simulink model "SF009A_DutyCycThermProtn"  (R2013b)
settings: Solver=FixedStepDiscrete  SolverMode=SingleTasking  StartTime=0.0  StopTime=1  FixedStep=0.1  RelTol=1e-3
undefined symbols (not defined in the file): AbsltTThermLimCnt, ARCHGLBPRM_100MILLISEC_SEC_F32, CTRLRANDCUTFLT_CNT_U08, CTRLRTFLT_CNT_U08, CUTFLT_CNT_U08, DITHERMLIM_MOTNWTMTR_F32, DutyCycExcddCnt, DutyCycThermProtnAbsltCtrlTTblX, DutyCycThermProtnAbsltCtrlTTqTblY, DutyCycThermProtnAbsltCuTTblX, DutyCycThermProtnAbsltCuTTqTblY, DutyCycThermProtnAbsltMotVelBreakPt, DutyCycThermProtnAbsltTTqSlewHiLim, DutyCycThermProtnAbsltTTqSlewLoLim, DutyCycThermProtnCtrlT, DutyCycThermProtnCtrlTSeln, DutyCycThermProtnDutyCycFildThd, DutyCycThermProtnIgnOffCtrlEna, DutyCycThermProtnIgnOffMsgWaitTi, DutyCycThermProtnLstTblValNonStall, DutyCycThermProtnLstTblValStall, DutyCycThermProtnMotPrTSeln, DutyCycThermProtnMplr1NonStallTblY, DutyCycThermProtnMplr1StallTblY, DutyCycThermProtnMplr2NonStallTblY, DutyCycThermProtnMplr2StallTblY, DutyCycThermProtnMplr3NonStallTblY, DutyCycThermProtnMplr3StallTblY, DutyCycThermProtnMplr4NonStallTblY, DutyCycThermProtnMplr4StallTblY, DutyCycThermProtnMplr5NonStallTblY, DutyCycThermProtnMplr5StallTblY, DutyCycThermProtnMplr6NonStallTblY, DutyCycThermProtnMplr6StallTblY, DutyCycThermProtnMplrTblX, DutyCycThermProtnMplrTSeln, DutyCycThermProtnSlowFilTSeln, DutyCycThermProtnThermLoadLimTblX, DutyCycThermProtnThermLoadLimTblY, DutyCycThermProtnTqCmdSlewDwn, DutyCycThermProtnTqCmdSlewUp, FILVALMIN_ULS_F32, IGNTIOFFTHD_CNT_F32, NODEBSTEP_CNT_U16, NtcSts1, NvmGetErrSts1, ONEPERC_ULS_F32, TAU3_SEC_F32, TAU4_SEC_F32, TAU5_SEC_F32, TAU6_SEC_F32, THERMLOADLIMTBLIDX_ULS_U08
libraries: FixdToFloat x13, Fil x12, simulink x11, NxtrLim x10, NxtrMath x8, FloatToFixd x6, NxtrMax x6, NxtrMin x4, NxtrAbslt x2, NxtrNvM x1
(part 3 of 6)

== system SF009A_DutyCycThermProtn/DutyCycThermProtn/DutyCycThermProtnInit1/PowerOnTasks/DefaultIgnOffTime ==
  Action Port : ActionPort  ActionType=else
  CopyRight2 : Subsystem  Description=|  mask(Copyright Information){none=on}
      | Copyright info block.                                               
      |                                                                     
      | Place copyright information at the top of every subsystem in design.
      mask prompts: none "No parameters"
      mask help: Place copyright information at the top of every subsystem in design.
      mask Display:
      | NxtrConf = 'Nexteer Confidential';
      | 
      | sys = bdroot; %handle for the current model ("system")
      | first = get_param(sys,'Created');
      | first = first(end-3:end);  %year is last four digits
      | 
      | last = get_param(sys,'LastModifiedDate');
      | if isempty(last)
      |     last = datestr(now,'yyyy');
      | else
      |     last = last(end-3:end);
      | end
      | 
      | if strcmp(first,last)
      |     fprintf('%s -- Copyright %s Nexteer',NxtrConf,first)
      | else
      |     fprintf('%s -- %s%s- %s Nexteer',NxtrConf,char(169),first,last)
      | end
  DefIgnOffTime1 : Constant  RequirementInfo="{'linktype_rmi_doors' '0000a52a (/E-STEER Core/SubSystem Specifications/Application Functions/SF009A Thermal Duty Cycle Protection)' '#SF009A_285' 'true' 'REQ:  SF009A_285' '' } %GIDa_1c1a8355_68c4_4a16_a698_2c7b860aa81f"  Value=FILVALMIN_ULS_F32
  FiltSV3 : Outport  RequirementInfo="{'linktype_rmi_doors' '0000a52a (/E-STEER Core/SubSystem Specifications/Application Functions/SF009A Thermal Duty Cycle Protection)' '#SF009A_285' 'true' 'REQ:  SF009A_285' '' } %GIDa_f53f9a1c_8faf_4833_a80c_e2891c436a6f"
  FiltSV4 : Outport  RequirementInfo="{'linktype_rmi_doors' '0000a52a (/E-STEER Core/SubSystem Specifications/Application Functions/SF009A Thermal Duty Cycle Protection)' '#SF009A_285' 'true' 'REQ:  SF009A_285' '' } %GIDa_7573da05_c607_444c_bff7_05b9be356769"  Port=2
  FiltSV5 : Outport  RequirementInfo="{'linktype_rmi_doors' '0000a52a (/E-STEER Core/SubSystem Specifications/Application Functions/SF009A Thermal Duty Cycle Protection)' '#SF009A_285' 'true' 'REQ:  SF009A_285' '' } %GIDa_0a22d052_a9b5_4254_83f4_8f154e55c7ba"  Port=3
  FiltSV6 : Outport  RequirementInfo="{'linktype_rmi_doors' '0000a52a (/E-STEER Core/SubSystem Specifications/Application Functions/SF009A Thermal Duty Cycle Protection)' '#SF009A_285' 'true' 'REQ:  SF009A_285' '' } %GIDa_7f0b1c6f_6523_47e0_8553_42c05ca6b0db"  Port=4
  wires:
  DefIgnOffTime1/1 -> FiltSV3/1, FiltSV4/1, FiltSV6/1, FiltSV5/1

== system SF009A_DutyCycThermProtn/DutyCycThermProtn/DutyCycThermProtnInit1/PowerOnTasks/InputIgnOffTime ==
  note: RANGE CHECK, ENSURE VALUE IS BELOW A CONSTANT (10000)
  IgnTiOff : Inport
  Action Port : ActionPort  ActionType=then
  CopyRight2 : Subsystem  Description=|  mask(Copyright Information){none=on}
      | Copyright info block.                                               
      |                                                                     
      | Place copyright information at the top of every subsystem in design.
      mask prompts: none "No parameters"
      mask help: Place copyright information at the top of every subsystem in design.
      mask Display:
      | NxtrConf = 'Nexteer Confidential';
      | 
      | sys = bdroot; %handle for the current model ("system")
      | first = get_param(sys,'Created');
      | first = first(end-3:end);  %year is last four digits
      | 
      | last = get_param(sys,'LastModifiedDate');
      | if isempty(last)
      |     last = datestr(now,'yyyy');
      | else
      |     last = last(end-3:end);
      | end
      | 
      | if strcmp(first,last)
      |     fprintf('%s -- Copyright %s Nexteer',NxtrConf,first)
      | else
      |     fprintf('%s -- %s%s- %s Nexteer',NxtrConf,char(169),first,last)
      | end
  Data Store Read : DataStoreRead  DataStoreName=FilStVal  DataStoreElements=FilStVal.Fil3StVal
  Data Store Read1 : DataStoreRead  DataStoreName=FilStVal  DataStoreElements=FilStVal.Fil4StVal
  Data Store Read2 : DataStoreRead  DataStoreName=FilStVal  DataStoreElements=FilStVal.Fil5StVal
  Data Store Read3 : DataStoreRead  DataStoreName=FilStVal  DataStoreElements=FilStVal.Fil6StVal
  Filt3ExpDecay : Subsystem  RequirementInfo={} %GIDa_9f9f3f65_c145_44e4_82e5_fd713760ae68
  Filt4ExpDecay : Subsystem  RequirementInfo={} %GIDa_626963e8_8ecf_441f_b1c9_4240579d77f9
  Filt5ExpDecay : Subsystem  RequirementInfo={} %GIDa_9364c89b_18fa_4473_8499_21374c540da9
  Filt6ExpDecay : Subsystem  RequirementInfo={} %GIDa_8e6049b9_bd81_40a5_96f3_6037c184dcb3
  FiltSV3 : Outport
  FiltSV4 : Outport  Port=2
  FiltSV5 : Outport  Port=3
  FiltSV6 : Outport  Port=4
  wires:
  Filt3ExpDecay/1(FiltSV) -> FiltSV3/1
  Data Store Read/1 -> Filt3ExpDecay/2(FiltSVOrg)
  Filt4ExpDecay/1(FiltSV) -> FiltSV4/1
  Filt5ExpDecay/1(FiltSV) -> FiltSV5/1
  Data Store Read2/1 -> Filt5ExpDecay/2(FiltSVOrg)
  Filt6ExpDecay/1(FiltSV) -> FiltSV6/1
  Data Store Read3/1 -> Filt6ExpDecay/2(FiltSVOrg)
  Data Store Read1/1 -> Filt4ExpDecay/2(FiltSVOrg)
  IgnTiOff/1 -> Filt3ExpDecay/1(IgnTimeOffSel), Filt4ExpDecay/1(IgnTimeOffSel), Filt6ExpDecay/1(IgnTimeOffSel), Filt5ExpDecay/1(IgnTimeOffSel)

== system SF009A_DutyCycThermProtn/DutyCycThermProtn/DutyCycThermProtnInit1/SetInitialValueOfAbsTempLimitSlew/Copyright1 ==

== system SF009A_DutyCycThermProtn/DutyCycThermProtn/DutyCycThermProtnInit1/SetInitialValueOfLstTblValRateLimrStVari/Copyright1 ==

== system SF009A_DutyCycThermProtn/DutyCycThermProtn/DutyCycThermProtnPer1/FiltSVReinit/CopyRight2 ==

== system SF009A_DutyCycThermProtn/DutyCycThermProtn/DutyCycThermProtnPer1/FiltSVReinit/VehTiVldDisabled ==
  Action Port : ActionPort  ActionType=else
  CopyRight2 : Subsystem  Description=|  mask(Copyright Information){none=on}
      | Copyright info block.                                               
      |                                                                     
      | Place copyright information at the top of every subsystem in design.
      mask prompts: none "No parameters"
      mask help: Place copyright information at the top of every subsystem in design.
      mask Display:
      | NxtrConf = 'Nexteer Confidential';
      | 
      | sys = bdroot; %handle for the current model ("system")
      | first = get_param(sys,'Created');
      | first = first(end-3:end);  %year is last four digits
      | 
      | last = get_param(sys,'LastModifiedDate');
      | if isempty(last)
      |     last = datestr(now,'yyyy');
      | else
      |     last = last(end-3:end);
      | end
      | 
      | if strcmp(first,last)
      |     fprintf('%s -- Copyright %s Nexteer',NxtrConf,first)
      | else
      |     fprintf('%s -- %s%s- %s Nexteer',NxtrConf,char(169),first,last)
      | end
  DefIgnOffTime1 : Constant  RequirementInfo="{'linktype_rmi_doors' '0000a52a (/E-STEER Core/SubSystem Specifications/Application Functions/SF009A Thermal Duty Cycle Protection)' '#SF009A_285' 'true' 'REQ:  SF009A_285' '' } %GIDa_ff571b1a_1782_4f5b_8061_ceec6519b3d1"  Value=FILVALMIN_ULS_F32
  FiltSV3 : Outport  RequirementInfo="{'linktype_rmi_doors' '0000a52a (/E-STEER Core/SubSystem Specifications/Application Functions/SF009A Thermal Duty Cycle Protection)' '#SF009A_285' 'true' 'REQ:  SF009A_285' '' } %GIDa_7dd21f81_ccc7_49b6_9939_90cfad62de91"
  FiltSV4 : Outport  RequirementInfo="{'linktype_rmi_doors' '0000a52a (/E-STEER Core/SubSystem Specifications/Application Functions/SF009A Thermal Duty Cycle Protection)' '#SF009A_285' 'true' 'REQ:  SF009A_285' '' } %GIDa_9e3d7e87_4137_4c20_943f_e98c68156777"  Port=2
  FiltSV5 : Outport  RequirementInfo="{'linktype_rmi_doors' '0000a52a (/E-STEER Core/SubSystem Specifications/Application Functions/SF009A Thermal Duty Cycle Protection)' '#SF009A_285' 'true' 'REQ:  SF009A_285' '' } %GIDa_7d2d2855_4602_487a_979b_6bffe0216b93"  Port=3
  FiltSV6 : Outport  RequirementInfo="{'linktype_rmi_doors' '0000a52a (/E-STEER Core/SubSystem Specifications/Application Functions/SF009A Thermal Duty Cycle Protection)' '#SF009A_285' 'true' 'REQ:  SF009A_285' '' } %GIDa_d4f64410_e786_41b0_841d_daea9815ca41"  Port=4
  wires:
  DefIgnOffTime1/1 -> FiltSV3/1, FiltSV4/1, FiltSV6/1, FiltSV5/1

== system SF009A_DutyCycThermProtn/DutyCycThermProtn/DutyCycThermProtnPer1/FiltSVReinit/VehTiVldEnabled ==
  IgnTiOff : Inport
  Action Port : ActionPort  ActionType=then
  CopyRight2 : Subsystem  Description=|  mask(Copyright Information){none=on}
      | Copyright info block.                                               
      |                                                                     
      | Place copyright information at the top of every subsystem in design.
      mask prompts: none "No parameters"
      mask help: Place copyright information at the top of every subsystem in design.
      mask Display:
      | NxtrConf = 'Nexteer Confidential';
      | 
      | sys = bdroot; %handle for the current model ("system")
      | first = get_param(sys,'Created');
      | first = first(end-3:end);  %year is last four digits
      | 
      | last = get_param(sys,'LastModifiedDate');
      | if isempty(last)
      |     last = datestr(now,'yyyy');
      | else
      |     last = last(end-3:end);
      | end
      | 
      | if strcmp(first,last)
      |     fprintf('%s -- Copyright %s Nexteer',NxtrConf,first)
      | else
      |     fprintf('%s -- %s%s- %s Nexteer',NxtrConf,char(169),first,last)
      | end
  Data Store Read : DataStoreRead  DataStoreName=Fil3ValPwrUp
  Data Store Read1 : DataStoreRead  DataStoreName=Fil4ValPwrUp
  Data Store Read2 : DataStoreRead  DataStoreName=Fil5ValPwrUp
  Data Store Read3 : DataStoreRead  DataStoreName=Fil6ValPwrUp
  Filt3ExpDecay : Subsystem
  Filt4ExpDecay : Subsystem
  Filt5ExpDecay : Subsystem
  Filt6ExpDecay : Subsystem
  FiltSV3 : Outport
  FiltSV4 : Outport  Port=2
  FiltSV5 : Outport  Port=3
  FiltSV6 : Outport  Port=4
  wires:
  IgnTiOff/1 -> Filt6ExpDecay/1(IgnTimeOffSel), Filt5ExpDecay/1(IgnTimeOffSel), Filt4ExpDecay/1(IgnTimeOffSel), Filt3ExpDecay/1(IgnTimeOffSel)
  Data Store Read3/1 -> Filt6ExpDecay/2(FiltSVOrg)
  Filt6ExpDecay/1(FiltSV) -> FiltSV6/1
  Data Store Read2/1 -> Filt5ExpDecay/2(FiltSVOrg)
  Filt5ExpDecay/1(FiltSV) -> FiltSV5/1
  Data Store Read1/1 -> Filt4ExpDecay/2(FiltSVOrg)
  Filt4ExpDecay/1(FiltSV) -> FiltSV4/1
  Data Store Read/1 -> Filt3ExpDecay/2(FiltSVOrg)
  Filt3ExpDecay/1(FiltSV) -> FiltSV3/1

== system SF009A_DutyCycThermProtn/DutyCycThermProtn/DutyCycThermProtnPer1/LoadLimiting/CopyRight2 ==

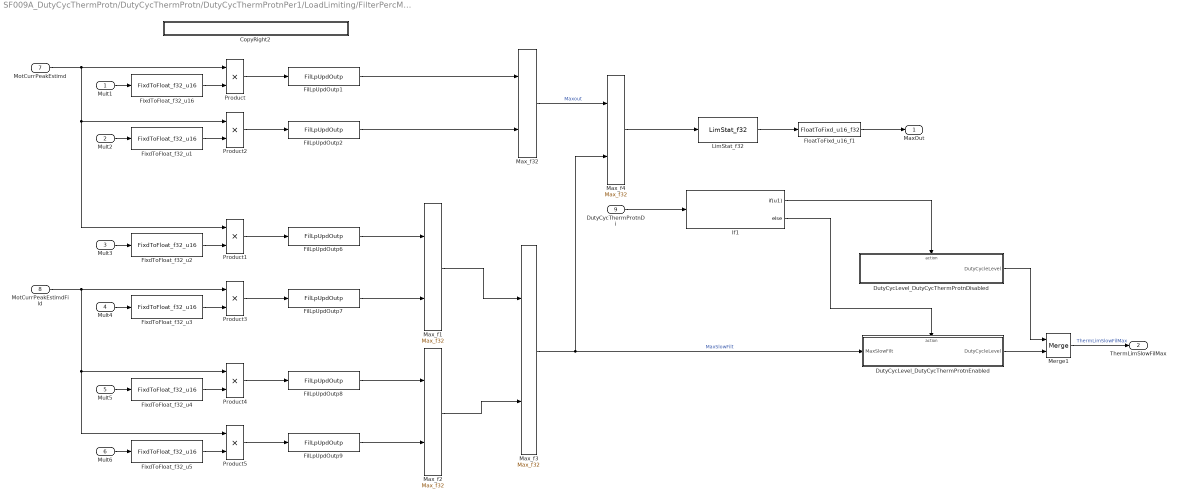
== system SF009A_DutyCycThermProtn/DutyCycThermProtn/DutyCycThermProtnPer1/LoadLimiting/FilterPercMax ==
  Mult1 : Inport
  Mult2 : Inport  Port=2
  Mult3 : Inport  Port=3
  Mult4 : Inport  Port=4
  Mult5 : Inport  Port=5
  Mult6 : Inport  Port=6
  MotCurrPeakEstimd : Inport  Port=7
  MotCurrPeakEstimdFild : Inport  Port=8
  DutyCycThermProtnDi : Inport  Port=9
  CopyRight2 : Subsystem  Description=|  mask(Copyright Information){none=on}
      | Copyright info block.                                               
      |                                                                     
      | Place copyright information at the top of every subsystem in design.
      mask prompts: none "No parameters"
      mask help: Place copyright information at the top of every subsystem in design.
      mask Display:
      | NxtrConf = 'Nexteer Confidential';
      | 
      | sys = bdroot; %handle for the current model ("system")
      | first = get_param(sys,'Created');
      | first = first(end-3:end);  %year is last four digits
      | 
      | last = get_param(sys,'LastModifiedDate');
      | if isempty(last)
      |     last = datestr(now,'yyyy');
      | else
      |     last = last(end-3:end);
      | end
      | 
      | if strcmp(first,last)
      |     fprintf('%s -- Copyright %s Nexteer',NxtrConf,first)
      | else
      |     fprintf('%s -- %s%s- %s Nexteer',NxtrConf,char(169),first,last)
      | end
  DutyCycLevel_DutyCycThermProtnDisabled : Subsystem  RequirementInfo="{'linktype_rmi_doors' '0000a52a (/E-STEER Core/SubSystem Specifications/Application Functions/SF009A Thermal Duty Cycle Protection)' '#SF009A_168' 'true' 'REQ:  SF009A_168' '' } %GIDa_71363024_cb12_46dd_971c_3c161e9d529d"  TreatAsAtomicUnit=on
  DutyCycLevel_DutyCycThermProtnEnabled : Subsystem  RequirementInfo="{'linktype_rmi_doors' '0000a52a (/E-STEER Core/SubSystem Specifications/Application Functions/SF009A Thermal Duty Cycle Protection)' '#SF009A_168' 'true' 'REQ:  SF009A_168' '' } %GIDa_1862e0cc_48c0_4a64_b3aa_9ef2fa11f229"  TreatAsAtomicUnit=on
  FilLpUpdOutp1 : Fil/FilLpUpdOutp  RequirementInfo="{'linktype_rmi_doors' '0000a52a (/E-STEER Core/SubSystem Specifications/Application Functions/SF009A Thermal Duty Cycle Protection)' '#SF009A_117' 'true' 'REQ:  SF009A_117' '' } %GIDa_36d69916_80a2_4684_8052_fd4d54618007"  StVar=Fil1ValStVari
      settings: AttributesFormatString=StVar: %<StVar>
  FilLpUpdOutp2 : Fil/FilLpUpdOutp  RequirementInfo="{'linktype_rmi_doors' '0000a52a (/E-STEER Core/SubSystem Specifications/Application Functions/SF009A Thermal Duty Cycle Protection)' '#SF009A_117' 'true' 'REQ:  SF009A_117' '' } %GIDa_9334f7f9_570f_473a_a841_bd6f3c21f9df"  StVar=Fil2ValStVari
      settings: AttributesFormatString=StVar: %<StVar>
  FilLpUpdOutp6 : Fil/FilLpUpdOutp  RequirementInfo="{'linktype_rmi_doors' '0000a52a (/E-STEER Core/SubSystem Specifications/Application Functions/SF009A Thermal Duty Cycle Protection)' '#SF009A_117' 'true' 'REQ:  SF009A_117' '' } %GIDa_8cd640f7_4fe0_46fd_98bb_13b2eab9fb91"  StVar=Fild3Val
      settings: AttributesFormatString=StVar: %<StVar>
  FilLpUpdOutp7 : Fil/FilLpUpdOutp  RequirementInfo="{'linktype_rmi_doors' '0000a52a (/E-STEER Core/SubSystem Specifications/Application Functions/SF009A Thermal Duty Cycle Protection)' '#SF009A_117' 'true' 'REQ:  SF009A_117' '' } %GIDa_84154e02_2e1c_41ac_9811_25a1fbb85ef4"  StVar=Fild4Val
      settings: AttributesFormatString=StVar: %<StVar>
  FilLpUpdOutp8 : Fil/FilLpUpdOutp  RequirementInfo="{'linktype_rmi_doors' '0000a52a (/E-STEER Core/SubSystem Specifications/Application Functions/SF009A Thermal Duty Cycle Protection)' '#SF009A_117' 'true' 'REQ:  SF009A_117' '' } %GIDa_4a9913a0_954a_4382_b1cf_522ede446f9f"  StVar=Fild5Val
      settings: AttributesFormatString=StVar: %<StVar>
  FilLpUpdOutp9 : Fil/FilLpUpdOutp  RequirementInfo="{'linktype_rmi_doors' '0000a52a (/E-STEER Core/SubSystem Specifications/Application Functions/SF009A Thermal Duty Cycle Protection)' '#SF009A_117' 'true' 'REQ:  SF009A_117' '' } %GIDa_c55f5e10_5865_48ee_8ffc_2f75da5ed5de"  StVar=Fild6Val
      settings: AttributesFormatString=StVar: %<StVar>
  FixdToFloat_f32_u{1..5,16} (6 alike) : FixdToFloat/FixdToFloat_f32_u16  Param1=13
  FloatToFixd_u16_f1 : FloatToFixd/FloatToFixd_u16_f32  Param1=0
  If1 : If  RequirementInfo="{'linktype_rmi_doors' '0000a52a (/E-STEER Core/SubSystem Specifications/Application Functions/SF009A Thermal Duty Cycle Protection)' '#SF009A_168' 'true' 'REQ:  SF009A_168' '' } %GIDa_157cb9dd_8c28_4ea7_a2f6_9f40ccd5ede0"  IfExpression=u1
  LimStat_f32 : NxtrLim/LimStat_f32  LoLim=single(0)  HiLim=FILOUTPLIM_ULS_F32
      settings: AttributesFormatString=Lower Limit: %<LoLim>\nUpper Limit: %<HiLim>
  Max_f1 : NxtrMax/Max_f32  RequirementInfo="{'linktype_rmi_doors' '0000a52a (/E-STEER Core/SubSystem Specifications/Application Functions/SF009A Thermal Duty Cycle Protection)' '#SF009A_164' 'true' 'REQ:  SF009A_164' '' ; 'linktype_rmi_doors' '0000a52a (/E-STEER Core/SubSystem Specifications/Application Functions/SF009A Thermal Duty Cycle Protection)' '#SF009A_167' 'true' 'REQ:  SF009A_167' '' } %GIDa_ca8925de_f515_4e09_b430_d40efee02347"  SFunctionSpec=single y1 = Max_f32(single u1, single u2)
  Max_f2 : NxtrMax/Max_f32  RequirementInfo="{'linktype_rmi_doors' '0000a52a (/E-STEER Core/SubSystem Specifications/Application Functions/SF009A Thermal Duty Cycle Protection)' '#SF009A_164' 'true' 'REQ:  SF009A_164' '' ; 'linktype_rmi_doors' '0000a52a (/E-STEER Core/SubSystem Specifications/Application Functions/SF009A Thermal Duty Cycle Protection)' '#SF009A_167' 'true' 'REQ:  SF009A_167' '' } %GIDa_b559abac_2e26_4623_b247_6a9c382bd671"  SFunctionSpec=single y1 = Max_f32(single u1, single u2)
  Max_f3 : NxtrMax/Max_f32  RequirementInfo="{'linktype_rmi_doors' '0000a52a (/E-STEER Core/SubSystem Specifications/Application Functions/SF009A Thermal Duty Cycle Protection)' '#SF009A_164' 'true' 'REQ:  SF009A_164' '' ; 'linktype_rmi_doors' '0000a52a (/E-STEER Core/SubSystem Specifications/Application Functions/SF009A Thermal Duty Cycle Protection)' '#SF009A_167' 'true' 'REQ:  SF009A_167' '' } %GIDa_092cd743_3616_45d9_acc8_4304d3de2e74"  SFunctionSpec=single y1 = Max_f32(single u1, single u2)
  Max_f32 : NxtrMax/Max_f32  RequirementInfo="{'linktype_rmi_doors' '0000a52a (/E-STEER Core/SubSystem Specifications/Application Functions/SF009A Thermal Duty Cycle Protection)' '#SF009A_164' 'true' 'REQ:  SF009A_164' '' } %GIDa_d19587f6_c498_4d64_88b0_72feb27fc8ad"  SFunctionSpec=single y1 = Max_f32(single u1, single u2)
  Max_f4 : NxtrMax/Max_f32  RequirementInfo="{'linktype_rmi_doors' '0000a52a (/E-STEER Core/SubSystem Specifications/Application Functions/SF009A Thermal Duty Cycle Protection)' '#SF009A_164' 'true' 'REQ:  SF009A_164' '' } %GIDa_8231735f_1900_427b_8d69_95be75866dae"  SFunctionSpec=single y1 = Max_f32(single u1, single u2)
  Merge1 : Merge  RequirementInfo="{'linktype_rmi_doors' '0000a52a (/E-STEER Core/SubSystem Specifications/Application Functions/SF009A Thermal Duty Cycle Protection)' '#SF009A_168' 'true' 'REQ:  SF009A_168' '' } %GIDa_7470e7ba_5e3d_450c_abd9_7a59ae4fb17e"
  Product{,1..5} (6 alike) : Product  RndMeth=Zero
  MaxOut : Outport
  ThermLimSlowFilMax : Outport  RequirementInfo="{'linktype_rmi_doors' '0000a52a (/E-STEER Core/SubSystem Specifications/Application Functions/SF009A Thermal Duty Cycle Protection)' '#SF009A_257' 'true' 'REQ:  SF009A_257' '' } %GIDa_486bc804_3010_4761_b204_bb6960c359d5"  Port=2
  wires:
  FilLpUpdOutp6/1 -> Max_f1/1
  Max_f1/1 -> Max_f3/1
  LimStat_f32/1 -> FloatToFixd_u16_f1/1
  FilLpUpdOutp7/1 -> Max_f1/2
  FilLpUpdOutp8/1 -> Max_f2/1
  FilLpUpdOutp9/1 -> Max_f2/2
  Merge1/1 -> ThermLimSlowFilMax/1  "ThermLimSlowFilMax"
  MotCurrPeakEstimd/1 -> Product2/1, Product1/1, Product/1
  Mult1/1 -> FixdToFloat_f32_u16/1
  Mult3/1 -> FixdToFloat_f32_u2/1
  Mult2/1 -> FixdToFloat_f32_u1/1
  Product/1 -> FilLpUpdOutp1/1
  MotCurrPeakEstimdFild/1 -> Product3/1, Product5/1, Product4/1
  Mult4/1 -> FixdToFloat_f32_u3/1
  Mult5/1 -> FixdToFloat_f32_u4/1
  Mult6/1 -> FixdToFloat_f32_u5/1
  Product2/1 -> FilLpUpdOutp2/1
  Product1/1 -> FilLpUpdOutp6/1
  Product3/1 -> FilLpUpdOutp7/1
  Product4/1 -> FilLpUpdOutp8/1
  Product5/1 -> FilLpUpdOutp9/1
  FilLpUpdOutp1/1 -> Max_f32/1
  FilLpUpdOutp2/1 -> Max_f32/2
  DutyCycThermProtnDi/1 -> If1/1
  DutyCycLevel_DutyCycThermProtnDisabled/1(DutyCycleLevel) -> Merge1/1
  DutyCycLevel_DutyCycThermProtnEnabled/1(DutyCycleLevel) -> Merge1/2
  Max_f4/1 -> LimStat_f32/1
  If1/1 -> DutyCycLevel_DutyCycThermProtnDisabled/Action
  If1/2 -> DutyCycLevel_DutyCycThermProtnEnabled/Action
  Max_f2/1 -> Max_f3/2
  Max_f3/1 -> DutyCycLevel_DutyCycThermProtnEnabled/1(MaxSlowFilt), Max_f4/2  "MaxSlowFilt"
  Max_f32/1 -> Max_f4/1  "Maxout"
  FixdToFloat_f32_u16/1 -> Product/2
  FixdToFloat_f32_u1/1 -> Product2/2
  FixdToFloat_f32_u2/1 -> Product1/2
  FixdToFloat_f32_u3/1 -> Product3/2
  FixdToFloat_f32_u4/1 -> Product4/2
  FixdToFloat_f32_u5/1 -> Product5/2
  FloatToFixd_u16_f1/1 -> MaxOut/1

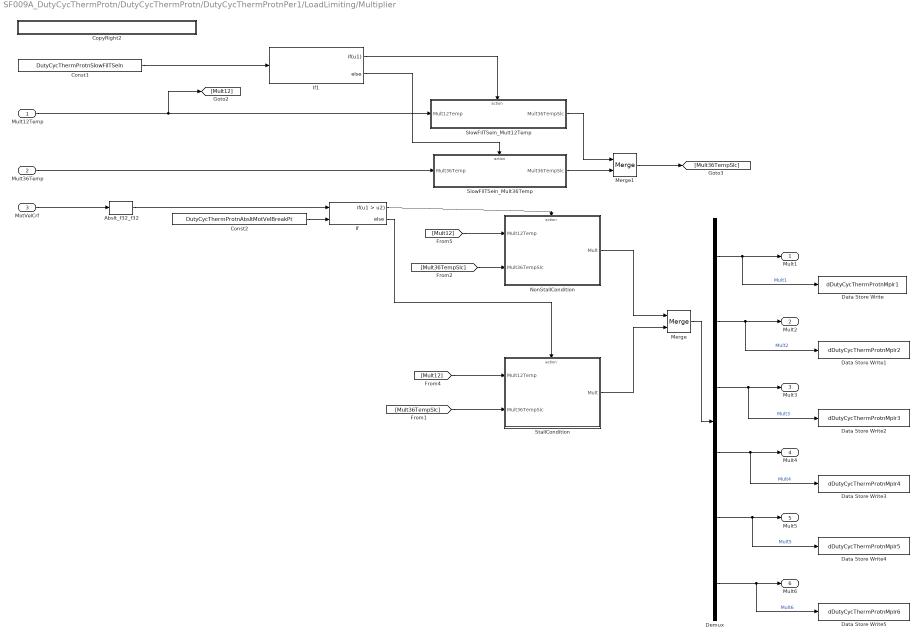
== system SF009A_DutyCycThermProtn/DutyCycThermProtn/DutyCycThermProtnPer1/LoadLimiting/Multiplier ==
  Mult12Temp : Inport
  Mult36Temp : Inport  Port=2
  MotVelCrf : Inport  Port=3
  Abslt_f32_f32 : NxtrAbslt/Abslt_f32_f32  SFunctionSpec=single y1 = Abslt_f32_f32(single u1)
      settings: AttributesFormatString=%<Name>
  Const1 : Constant  RequirementInfo="{'linktype_rmi_doors' '0000a52a (/E-STEER Core/SubSystem Specifications/Application Functions/SF009A Thermal Duty Cycle Protection)' '#SF009A_151' 'true' 'REQ:  SF009A_151' '' } %GIDa_87016093_dca7_4680_b392_3511aa636729"  Value=DutyCycThermProtnSlowFilTSeln
  Const2 : Constant  RequirementInfo="{'linktype_rmi_doors' '0000a52a (/E-STEER Core/SubSystem Specifications/Application Functions/SF009A Thermal Duty Cycle Protection)' '#SF009A_217' 'true' 'REQ:  SF009A_217' '' } %GIDa_e07e7f93_d6c7_47ef_bf2e_19c09e4ab3f5"  Value=DutyCycThermProtnAbsltMotVelBreakPt
  CopyRight2 : Subsystem  Description=|  mask(Copyright Information){none=on}
      | Copyright info block.                                               
      |                                                                     
      | Place copyright information at the top of every subsystem in design.
      mask prompts: none "No parameters"
      mask help: Place copyright information at the top of every subsystem in design.
      mask Display:
      | NxtrConf = 'Nexteer Confidential';
      | 
      | sys = bdroot; %handle for the current model ("system")
      | first = get_param(sys,'Created');
      | first = first(end-3:end);  %year is last four digits
      | 
      | last = get_param(sys,'LastModifiedDate');
      | if isempty(last)
      |     last = datestr(now,'yyyy');
      | else
      |     last = last(end-3:end);
      | end
      | 
      | if strcmp(first,last)
      |     fprintf('%s -- Copyright %s Nexteer',NxtrConf,first)
      | else
      |     fprintf('%s -- %s%s- %s Nexteer',NxtrConf,char(169),first,last)
      | end
  Data Store Write : DataStoreWrite  DataStoreName=dDutyCycThermProtnMplr1
  Data Store Write1 : DataStoreWrite  DataStoreName=dDutyCycThermProtnMplr2
  Data Store Write2 : DataStoreWrite  DataStoreName=dDutyCycThermProtnMplr3
  Data Store Write3 : DataStoreWrite  DataStoreName=dDutyCycThermProtnMplr4
  Data Store Write4 : DataStoreWrite  DataStoreName=dDutyCycThermProtnMplr5
  Data Store Write5 : DataStoreWrite  DataStoreName=dDutyCycThermProtnMplr6
  Demux : Demux  Outputs=6
  If : If  RequirementInfo="{'linktype_rmi_doors' '0000a52a (/E-STEER Core/SubSystem Specifications/Application Functions/SF009A Thermal Duty Cycle Protection)' '#SF009A_116' 'true' 'REQ:  SF009A_116' '' } %GIDa_d0360e02_97ce_48cf_8672_eb1c09016105"  NumInputs=2  IfExpression=u1 > u2
  If1 : If  RequirementInfo="{'linktype_rmi_doors' '0000a52a (/E-STEER Core/SubSystem Specifications/Application Functions/SF009A Thermal Duty Cycle Protection)' '#SF009A_151' 'true' 'REQ:  SF009A_151' '' } %GIDa_2f381bbc_50d4_414d_93a6_c1ebc2063f26"  IfExpression=u1
  Merge : Merge  RequirementInfo="{'linktype_rmi_doors' '0000a52a (/E-STEER Core/SubSystem Specifications/Application Functions/SF009A Thermal Duty Cycle Protection)' '#SF009A_116' 'true' 'REQ:  SF009A_116' '' } %GIDa_424897de_be3d_4953_97de_501b9efc0782"
  Merge1 : Merge  RequirementInfo="{'linktype_rmi_doors' '0000a52a (/E-STEER Core/SubSystem Specifications/Application Functions/SF009A Thermal Duty Cycle Protection)' '#SF009A_151' 'true' 'REQ:  SF009A_151' '' } %GIDa_8d80e534_1858_41f5_a507_1f5b1fd28779"
  NonStallCondition : Subsystem  RequirementInfo="{'linktype_rmi_doors' '0000a52a (/E-STEER Core/SubSystem Specifications/Application Functions/SF009A Thermal Duty Cycle Protection)' '#SF009A_116' 'true' 'REQ:  SF009A_116' '' } %GIDa_c13999ff_915f_4750_b6af_90471e97e0b1"  TreatAsAtomicUnit=on
  SlowFilTSeln_Mult12Temp : Subsystem  RequirementInfo="{'linktype_rmi_doors' '0000a52a (/E-STEER Core/SubSystem Specifications/Application Functions/SF009A Thermal Duty Cycle Protection)' '#SF009A_151' 'true' 'REQ:  SF009A_151' '' } %GIDa_a6dc9a2e_a1d7_4331_9833_20d4c5c34ffd"  TreatAsAtomicUnit=on
  SlowFilTSeln_Mult36Temp : Subsystem  RequirementInfo="{'linktype_rmi_doors' '0000a52a (/E-STEER Core/SubSystem Specifications/Application Functions/SF009A Thermal Duty Cycle Protection)' '#SF009A_151' 'true' 'REQ:  SF009A_151' '' } %GIDa_6f859979_59ae_4faa_a03f_d836f73dc97e"  TreatAsAtomicUnit=on
  StallCondition : Subsystem  RequirementInfo="{'linktype_rmi_doors' '0000a52a (/E-STEER Core/SubSystem Specifications/Application Functions/SF009A Thermal Duty Cycle Protection)' '#SF009A_116' 'true' 'REQ:  SF009A_116' '' } %GIDa_1316cb19_780c_427c_a230_3bcb89e7d51b"  TreatAsAtomicUnit=on
  Mult1 : Outport  RequirementInfo="{'linktype_rmi_doors' '0000a52a (/E-STEER Core/SubSystem Specifications/Application Functions/SF009A Thermal Duty Cycle Protection)' '#SF009A_155' 'true' 'REQ:  SF009A_155' '' } %GIDa_fd8e61be_9bf0_4e18_a5e1_a43974329e69"
  Mult2 : Outport  RequirementInfo="{'linktype_rmi_doors' '0000a52a (/E-STEER Core/SubSystem Specifications/Application Functions/SF009A Thermal Duty Cycle Protection)' '#SF009A_155' 'true' 'REQ:  SF009A_155' '' } %GIDa_35190f10_f645_47f4_8361_57d755b725f3"  Port=2
  Mult3 : Outport  RequirementInfo="{'linktype_rmi_doors' '0000a52a (/E-STEER Core/SubSystem Specifications/Application Functions/SF009A Thermal Duty Cycle Protection)' '#SF009A_155' 'true' 'REQ:  SF009A_155' '' } %GIDa_c8fcc0c1_53bc_45d5_af25_a2bfad1812a3"  Port=3
  Mult4 : Outport  RequirementInfo="{'linktype_rmi_doors' '0000a52a (/E-STEER Core/SubSystem Specifications/Application Functions/SF009A Thermal Duty Cycle Protection)' '#SF009A_155' 'true' 'REQ:  SF009A_155' '' } %GIDa_954126f0_9343_400e_8331_66461f78390e"  Port=4
  Mult5 : Outport  RequirementInfo="{'linktype_rmi_doors' '0000a52a (/E-STEER Core/SubSystem Specifications/Application Functions/SF009A Thermal Duty Cycle Protection)' '#SF009A_155' 'true' 'REQ:  SF009A_155' '' } %GIDa_0c99cbdb_3a79_455c_847b_f10e0bf0b04c"  Port=5
  Mult6 : Outport  RequirementInfo="{'linktype_rmi_doors' '0000a52a (/E-STEER Core/SubSystem Specifications/Application Functions/SF009A Thermal Duty Cycle Protection)' '#SF009A_155' 'true' 'REQ:  SF009A_155' '' } %GIDa_13beb251_3ba5_4222_af48_e6cae6175380"  Port=6
  wires:
  Mult36Temp/1 -> SlowFilTSeln_Mult36Temp/1(Mult36Temp)
  Const1/1 -> If1/1
  MotVelCrf/1 -> Abslt_f32_f32/1
  Const2/1 -> If/2
  [Mult36TempSlc] -> NonStallCondition/2(Mult36TempSlc)
  Merge/1 -> Demux/1
  Demux/1 -> Data Store Write/1, Mult1/1  "Mult1"
  Demux/2 -> Data Store Write1/1, Mult2/1  "Mult2"
  Demux/3 -> Data Store Write2/1, Mult3/1  "Mult3"
  Demux/4 -> Data Store Write3/1, Mult4/1  "Mult4"
  Demux/5 -> Data Store Write4/1, Mult5/1  "Mult5"
  Demux/6 -> Data Store Write5/1, Mult6/1  "Mult6"
  Mult12Temp/1 -> [Mult12], SlowFilTSeln_Mult12Temp/1(Mult12Temp)
  [Mult12] -> NonStallCondition/1(Mult12Temp)
  Abslt_f32_f32/1 -> If/1
  [Mult36TempSlc] -> StallCondition/2(Mult36TempSlc)
  [Mult12] -> StallCondition/1(Mult12Temp)
  SlowFilTSeln_Mult12Temp/1(Mult36TempSlc) -> Merge1/1
  SlowFilTSeln_Mult36Temp/1(Mult36TempSlc) -> Merge1/2
  Merge1/1 -> [Mult36TempSlc]
  If1/1 -> SlowFilTSeln_Mult12Temp/Action
  If1/2 -> SlowFilTSeln_Mult36Temp/Action
  If/1 -> NonStallCondition/Action
  If/2 -> StallCondition/Action
  NonStallCondition/1(Mult) -> Merge/1
  StallCondition/1(Mult) -> Merge/2

== system SF009A_DutyCycThermProtn/DutyCycThermProtn/DutyCycThermProtnPer1/LoadLimiting/PowerOffTasks ==
  note: At power OFF, update NVM.
  CopyRight2 : Subsystem  Description=|  mask(Copyright Information){none=on}
      | Copyright info block.                                               
      |                                                                     
      | Place copyright information at the top of every subsystem in design.
      mask prompts: none "No parameters"
      mask help: Place copyright information at the top of every subsystem in design.
      mask Display:
      | NxtrConf = 'Nexteer Confidential';
      | 
      | sys = bdroot; %handle for the current model ("system")
      | first = get_param(sys,'Created');
      | first = first(end-3:end);  %year is last four digits
      | 
      | last = get_param(sys,'LastModifiedDate');
      | if isempty(last)
      |     last = datestr(now,'yyyy');
      | else
      |     last = last(end-3:end);
      | end
      | 
      | if strcmp(first,last)
      |     fprintf('%s -- Copyright %s Nexteer',NxtrConf,first)
      | else
      |     fprintf('%s -- %s%s- %s Nexteer',NxtrConf,char(169),first,last)
      | end
  Data Store Read1 : DataStoreRead  DataStoreName=Fild3Val  DataStoreElements=Fild3Val.FilSt
  Data Store Read2 : DataStoreRead  DataStoreName=Fild4Val  DataStoreElements=Fild4Val.FilSt
  Data Store Read3 : DataStoreRead  DataStoreName=Fild5Val  DataStoreElements=Fild5Val.FilSt
  Data Store Read4 : DataStoreRead  DataStoreName=Fild6Val  DataStoreElements=Fild6Val.FilSt
  Data Store Write : DataStoreWrite  DataStoreName=FilStVal  DataStoreElements=FilStVal.Fil3StVal
  Data Store Write1 : DataStoreWrite  DataStoreName=FilStVal  DataStoreElements=FilStVal.Fil4StVal
  Data Store Write2 : DataStoreWrite  DataStoreName=FilStVal  DataStoreElements=FilStVal.Fil5StVal
  Data Store Write3 : DataStoreWrite  DataStoreName=FilStVal  DataStoreElements=FilStVal.Fil6StVal
  Data Type Conversion{,1..3} (4 alike) : DataTypeConversion  OutDataTypeStr=uint8
  LimStat_f1 : NxtrLim/LimStat_f32  LoLim=FILVALMIN_ULS_F32  HiLim=FILVALMAX_ULS_F32
      settings: AttributesFormatString=Lower Limit: %<LoLim>\nUpper Limit: %<HiLim>
  LimStat_f2 : NxtrLim/LimStat_f32  LoLim=FILVALMIN_ULS_F32  HiLim=FILVALMAX_ULS_F32
      settings: AttributesFormatString=Lower Limit: %<LoLim>\nUpper Limit: %<HiLim>
  LimStat_f3 : NxtrLim/LimStat_f32  LoLim=FILVALMIN_ULS_F32  HiLim=FILVALMAX_ULS_F32
      settings: AttributesFormatString=Lower Limit: %<LoLim>\nUpper Limit: %<HiLim>
  LimStat_f32 : NxtrLim/LimStat_f32  RequirementInfo={} %GIDa_9cfebb92_a3ed_4173_aa17_612219a1860a  LoLim=FILVALMIN_ULS_F32  HiLim=FILVALMAX_ULS_F32
      settings: AttributesFormatString=Lower Limit: %<LoLim>\nUpper Limit: %<HiLim>
  wires:
  Data Store Read1/1 -> LimStat_f32/1
  LimStat_f32/1 -> Data Type Conversion/1
  LimStat_f1/1 -> Data Type Conversion1/1
  LimStat_f2/1 -> Data Type Conversion2/1
  LimStat_f3/1 -> Data Type Conversion3/1
  Data Store Read2/1 -> LimStat_f1/1
  Data Store Read3/1 -> LimStat_f2/1
  Data Store Read4/1 -> LimStat_f3/1
  Data Type Conversion/1 -> Data Store Write/1
  Data Type Conversion1/1 -> Data Store Write1/1
  Data Type Conversion2/1 -> Data Store Write2/1
  Data Type Conversion3/1 -> Data Store Write3/1

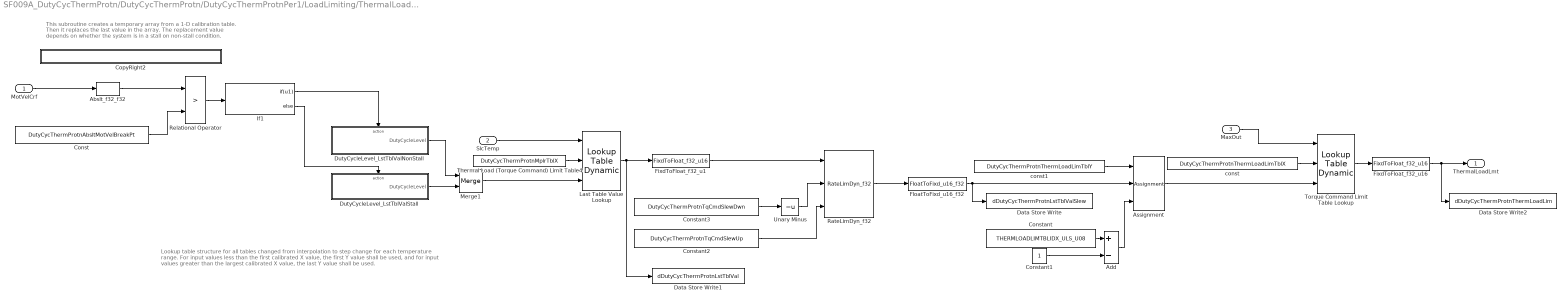
== system SF009A_DutyCycThermProtn/DutyCycThermProtn/DutyCycThermProtnPer1/LoadLimiting/ThermalLoadLimit ==
  note: Lookup table structure for all tables changed from interpolation to step change for each temperature range.
      | For input values less than the first calibrated X value, the first Y value shall be used, and for input values greater than the largest calibrated X value, the last Y value shall be used.
  note: This subroutine creates a temporary array from a 1-D calibration table.
      | Then it replaces the last value in the array. The replacement value
      | depends on whether the system is in a stall on non-stall condition.
  MotVelCrf : Inport
  SlcTemp : Inport  Port=2
  MaxOut : Inport  Port=3
  Abslt_f32_f32 : NxtrAbslt/Abslt_f32_f32  SFunctionSpec=single y1 = Abslt_f32_f32(single u1)
      settings: AttributesFormatString=%<Name>
  Add : Sum  Inputs=+-
  Assignment : Assignment  RequirementInfo="{'linktype_rmi_doors' '0000a52a (/E-STEER Core/SubSystem Specifications/Application Functions/SF009A Thermal Duty Cycle Protection)' '#SF009A_161' 'true' 'REQ:  SF009A_161' '' } %GIDa_1bfbba1b_7335_4ce6_8592_acc4710c3684"  IndexMode=Zero-based  IndexOptions=Index vector (port)  Indices=1  OutputSizes=1
  Const : Constant  RequirementInfo="{'linktype_rmi_doors' '0000a52a (/E-STEER Core/SubSystem Specifications/Application Functions/SF009A Thermal Duty Cycle Protection)' '#SF009A_213' 'true' 'REQ:  SF009A_213' '' } %GIDa_84ce6c55_5f14_483d_b925_fa849bec7b54"  Value=DutyCycThermProtnAbsltMotVelBreakPt
  Constant : Constant  Value=THERMLOADLIMTBLIDX_ULS_U08
  Constant1 : Constant  OutDataTypeStr=uint8
  Constant2 : Constant  RequirementInfo="{'linktype_rmi_doors' '0000a52a (/E-STEER Core/SubSystem Specifications/Application Functions/SF009A Thermal Duty Cycle Protection)' '#SF009A_162' 'true' 'REQ:  SF009A_162' '' } %GIDa_320606f8_aabd_4c85_b4ee_9fdcb7d69c3b"  Value=DutyCycThermProtnTqCmdSlewUp
  Constant3 : Constant  RequirementInfo="{'linktype_rmi_doors' '0000a52a (/E-STEER Core/SubSystem Specifications/Application Functions/SF009A Thermal Duty Cycle Protection)' '#SF009A_162' 'true' 'REQ:  SF009A_162' '' } %GIDa_e85aad03_ebd1_4ae2_9ef2_4862167cdcfb"  Value=DutyCycThermProtnTqCmdSlewDwn
  CopyRight2 : Subsystem  Description=|  mask(Copyright Information){none=on}
      | Copyright info block.                                               
      |                                                                     
      | Place copyright information at the top of every subsystem in design.
      mask prompts: none "No parameters"
      mask help: Place copyright information at the top of every subsystem in design.
      mask Display:
      | NxtrConf = 'Nexteer Confidential';
      | 
      | sys = bdroot; %handle for the current model ("system")
      | first = get_param(sys,'Created');
      | first = first(end-3:end);  %year is last four digits
      | 
      | last = get_param(sys,'LastModifiedDate');
      | if isempty(last)
      |     last = datestr(now,'yyyy');
      | else
      |     last = last(end-3:end);
      | end
      | 
      | if strcmp(first,last)
      |     fprintf('%s -- Copyright %s Nexteer',NxtrConf,first)
      | else
      |     fprintf('%s -- %s%s- %s Nexteer',NxtrConf,char(169),first,last)
      | end
  Data Store Write : DataStoreWrite  DataStoreName=dDutyCycThermProtnLstTblValSlew
  Data Store Write1 : DataStoreWrite  DataStoreName=dDutyCycThermProtnLstTblVal
  Data Store Write2 : DataStoreWrite  DataStoreName=dDutyCycThermProtnThermLoadLim
  DutyCycleLevel_LstTblValNonStall : Subsystem  RequirementInfo="{'linktype_rmi_doors' '0000a52a (/E-STEER Core/SubSystem Specifications/Application Functions/SF009A Thermal Duty Cycle Protection)' '#SF009A_213' 'true' 'REQ:  SF009A_213' '' } %GIDa_859b4a3f_9618_421c_8c12_ecc7c981f397"  TreatAsAtomicUnit=on
  DutyCycleLevel_LstTblValStall : Subsystem  RequirementInfo="{'linktype_rmi_doors' '0000a52a (/E-STEER Core/SubSystem Specifications/Application Functions/SF009A Thermal Duty Cycle Protection)' '#SF009A_213' 'true' 'REQ:  SF009A_213' '' } %GIDa_c9541d69_316c_47bc_a3b1_9dc8ba860312"  TreatAsAtomicUnit=on
  FixdToFloat_f32_u1 : FixdToFloat/FixdToFloat_f32_u16  Param1=7
  FixdToFloat_f32_u16 : FixdToFloat/FixdToFloat_f32_u16  Param1=7
  FloatToFixd_u16_f32 : FloatToFixd/FloatToFixd_u16_f32  Param1=7
  If1 : If  RequirementInfo="{'linktype_rmi_doors' '0000a52a (/E-STEER Core/SubSystem Specifications/Application Functions/SF009A Thermal Duty Cycle Protection)' '#SF009A_213' 'true' 'REQ:  SF009A_213' '' } %GIDa_996bb12d_37a0_42af_936a_bc51394247b8"  IfExpression=u1
  Last Table Value Lookup : simulink/Lookup Tables/Lookup Table Dynamic  RequirementInfo="{'linktype_rmi_doors' '0000a52a (/E-STEER Core/SubSystem Specifications/Application Functions/SF009A Thermal Duty Cycle Protection)' '#SF009A_214' 'true' 'REQ:  SF009A_214' '' ; 'linktype_rmi_doors' '0000a52a (/E-STEER Core/SubSystem Specifications/Application Functions/SF009A Thermal Duty Cycle Protection)' '#SF009A_166' 'true' 'REQ:  SF009A_166' '' } %GIDa_68fd95e5_e08d_4bd4_94f8_a3f7ad87c130"  LookUpMeth=Interpolation-Use End Values  OutDataTypeStr=Inherit: Inherit via back propagation  OutDataType=fixdt('double')  OutScaling=2^-10  DoSatur=off
  Merge1 : Merge  RequirementInfo="{'linktype_rmi_doors' '0000a52a (/E-STEER Core/SubSystem Specifications/Application Functions/SF009A Thermal Duty Cycle Protection)' '#SF009A_213' 'true' 'REQ:  SF009A_213' '' } %GIDa_f948dfcb_d0d2_4bd7_8081_3a80fecd33d9"
  RateLimDyn_f32 : NxtrLim/RateLimDyn_f32  RequirementInfo="{'linktype_rmi_doors' '0000a52a (/E-STEER Core/SubSystem Specifications/Application Functions/SF009A Thermal Duty Cycle Protection)' '#SF009A_162' 'true' 'REQ:  SF009A_162' '' } %GIDa_025d033f_00b9_4525_aacf_38dfba57462e"  StVar=LstTblValRateLimrStVari  Ts=ARCHGLBPRM_100MILLISEC_SEC_F32
      settings: AttributesFormatString=StVar: %<StVar>
  Relational Operator : RelationalOperator  RequirementInfo="{'linktype_rmi_doors' '0000a52a (/E-STEER Core/SubSystem Specifications/Application Functions/SF009A Thermal Duty Cycle Protection)' '#SF009A_213' 'true' 'REQ:  SF009A_213' '' } %GIDa_8a104490_fbca_4d73_ac9c_676f1690ad78"  Operator=>  OutDataTypeStr=boolean
  Thermal Load (Torque Command) Limit Table4 : Constant  RequirementInfo="{'linktype_rmi_doors' '0000a52a (/E-STEER Core/SubSystem Specifications/Application Functions/SF009A Thermal Duty Cycle Protection)' '#SF009A_214' 'true' 'REQ:  SF009A_214' '' } %GIDa_5b443c83_a5f2_454b_b43c_3081d53ced64"  Value=DutyCycThermProtnMplrTblX
  Torque Command Limit Table Lookup : simulink/Lookup Tables/Lookup Table Dynamic  RequirementInfo="{'linktype_rmi_doors' '0000a52a (/E-STEER Core/SubSystem Specifications/Application Functions/SF009A Thermal Duty Cycle Protection)' '#SF009A_263' 'true' 'REQ:  SF009A_263' '' } %GIDa_5c24fa18_10c0_4e86_9434_06f256897eb6"  LookUpMeth=Interpolation-Use End Values  OutDataTypeStr=Inherit: Inherit via back propagation  OutDataType=fixdt('double')  OutScaling=2^-10  DoSatur=off
  Unary Minus : UnaryMinus  RequirementInfo="{'linktype_rmi_doors' '0000a52a (/E-STEER Core/SubSystem Specifications/Application Functions/SF009A Thermal Duty Cycle Protection)' '#SF009A_162' 'true' 'REQ:  SF009A_162' '' } %GIDa_ab681b50_daa7_49c9_982e_0d084bf7f24a"
  const : Constant  RequirementInfo="{'linktype_rmi_doors' '0000a52a (/E-STEER Core/SubSystem Specifications/Application Functions/SF009A Thermal Duty Cycle Protection)' '#SF009A_215' 'true' 'REQ:  SF009A_215' '' } %GIDa_23cb79fa_b26f_403e_8875_b2b08b14118a"  Value=DutyCycThermProtnThermLoadLimTblX
  const1 : Constant  RequirementInfo="{'linktype_rmi_doors' '0000a52a (/E-STEER Core/SubSystem Specifications/Application Functions/SF009A Thermal Duty Cycle Protection)' '#SF009A_161' 'true' 'REQ:  SF009A_161' '' } %GIDa_93187d83_b3a0_45ad_ba61_f6dbc5effe25"  Value=DutyCycThermProtnThermLoadLimTblY
  ThermalLoadLmt : Outport
  wires:
  MotVelCrf/1 -> Abslt_f32_f32/1
  Const/1 -> Relational Operator/2
  Thermal Load (Torque Command) Limit Table4/1 -> Last Table Value Lookup/2
  Last Table Value Lookup/1 -> FixdToFloat_f32_u1/1, Data Store Write1/1
  Torque Command Limit Table Lookup/1 -> FixdToFloat_f32_u16/1
  Abslt_f32_f32/1 -> Relational Operator/1
  const/1 -> Torque Command Limit Table Lookup/2
  Merge1/1 -> Last Table Value Lookup/3
  DutyCycleLevel_LstTblValNonStall/1(DutyCycleLevel) -> Merge1/1
  DutyCycleLevel_LstTblValStall/1(DutyCycleLevel) -> Merge1/2
  Relational Operator/1 -> If1/1
  If1/1 -> DutyCycleLevel_LstTblValNonStall/Action
  If1/2 -> DutyCycleLevel_LstTblValStall/Action
  const1/1 -> Assignment/1
  Constant/1 -> Add/1
  SlcTemp/1 -> Last Table Value Lookup/1
  FixdToFloat_f32_u16/1 -> Data Store Write2/1, ThermalLoadLmt/1
  FloatToFixd_u16_f32/1 -> Assignment/2, Data Store Write/1
  FixdToFloat_f32_u1/1 -> RateLimDyn_f32/1
  Unary Minus/1 -> RateLimDyn_f32/2
  Constant3/1 -> Unary Minus/1
  Constant2/1 -> RateLimDyn_f32/3
  RateLimDyn_f32/1 -> FloatToFixd_u16_f32/1
  MaxOut/1 -> Torque Command Limit Table Lookup/1
  Assignment/1 -> Torque Command Limit Table Lookup/3
  Add/1 -> Assignment/3
  Constant1/1 -> Add/2

== system SF009A_DutyCycThermProtn/DutyCycThermProtn/DutyCycThermProtnPer1/ServiceDefeatFiltSVReinit/CopyRight2 ==

== system SF009A_DutyCycThermProtn/DutyCycThermProtn/DutyCycThermProtnPer1/TemperatureSelection/CopyRight2 ==

== system SF009A_DutyCycThermProtn/DutyCycThermProtn/DutyCycThermProtnPer1/TemperatureSelection/MplrTSelnDisabled ==
  Mult36Temp : Inport
  Action Port : ActionPort  ActionType=else
  CopyRight2 : Subsystem  Description=|  mask(Copyright Information){none=on}
      | Copyright info block.                                               
      |                                                                     
      | Place copyright information at the top of every subsystem in design.
      mask prompts: none "No parameters"
      mask help: Place copyright information at the top of every subsystem in design.
      mask Display:
      | NxtrConf = 'Nexteer Confidential';
      | 
      | sys = bdroot; %handle for the current model ("system")
      | first = get_param(sys,'Created');
      | first = first(end-3:end);  %year is last four digits
      | 
      | last = get_param(sys,'LastModifiedDate');
      | if isempty(last)
      |     last = datestr(now,'yyyy');
      | else
      |     last = last(end-3:end);
      | end
      | 
      | if strcmp(first,last)
      |     fprintf('%s -- Copyright %s Nexteer',NxtrConf,first)
      | else
      |     fprintf('%s -- %s%s- %s Nexteer',NxtrConf,char(169),first,last)
      | end
  SlcTemp : Outport
  wires:
  Mult36Temp/1 -> SlcTemp/1

== system SF009A_DutyCycThermProtn/DutyCycThermProtn/DutyCycThermProtnPer1/TemperatureSelection/MplrTSelnEnabled ==
  Mult12Temp : Inport
  Action Port : ActionPort  ActionType=then
  CopyRight2 : Subsystem  Description=|  mask(Copyright Information){none=on}
      | Copyright info block.                                               
      |                                                                     
      | Place copyright information at the top of every subsystem in design.
      mask prompts: none "No parameters"
      mask help: Place copyright information at the top of every subsystem in design.
      mask Display:
      | NxtrConf = 'Nexteer Confidential';
      | 
      | sys = bdroot; %handle for the current model ("system")
      | first = get_param(sys,'Created');
      | first = first(end-3:end);  %year is last four digits
      | 
      | last = get_param(sys,'LastModifiedDate');
      | if isempty(last)
      |     last = datestr(now,'yyyy');
      | else
      |     last = last(end-3:end);
      | end
      | 
      | if strcmp(first,last)
      |     fprintf('%s -- Copyright %s Nexteer',NxtrConf,first)
      | else
      |     fprintf('%s -- %s%s- %s Nexteer',NxtrConf,char(169),first,last)
      | end
  SlcTemp : Outport
  wires:
  Mult12Temp/1 -> SlcTemp/1

== system SF009A_DutyCycThermProtn/DutyCycThermProtn/DutyCycThermProtnPer1/TemperatureSelection/Mult12T_DiagcStsLimdTPrfmncDisabled ==
  EcuTFild : Inport
  MotFetT : Inport  Port=2
  Action Port : ActionPort  ActionType=else
  Calibration1 : Constant  RequirementInfo="{'linktype_rmi_doors' '0000a52a (/E-STEER Core/SubSystem Specifications/Application Functions/SF009A Thermal Duty Cycle Protection)' '#SF009A_113' 'true' 'REQ:  SF009A_113' '' } %GIDa_b6909ff9_455d_458d_8dc2_2b2011882908"  Value=DutyCycThermProtnCtrlTSeln
  CopyRight2 : Subsystem  Description=|  mask(Copyright Information){none=on}
      | Copyright info block.                                               
      |                                                                     
      | Place copyright information at the top of every subsystem in design.
      mask prompts: none "No parameters"
      mask help: Place copyright information at the top of every subsystem in design.
      mask Display:
      | NxtrConf = 'Nexteer Confidential';
      | 
      | sys = bdroot; %handle for the current model ("system")
      | first = get_param(sys,'Created');
      | first = first(end-3:end);  %year is last four digits
      | 
      | last = get_param(sys,'LastModifiedDate');
      | if isempty(last)
      |     last = datestr(now,'yyyy');
      | else
      |     last = last(end-3:end);
      | end
      | 
      | if strcmp(first,last)
      |     fprintf('%s -- Copyright %s Nexteer',NxtrConf,first)
      | else
      |     fprintf('%s -- %s%s- %s Nexteer',NxtrConf,char(169),first,last)
      | end
  CtrlTSelnDisabled : Subsystem  RequirementInfo="{'linktype_rmi_doors' '0000a52a (/E-STEER Core/SubSystem Specifications/Application Functions/SF009A Thermal Duty Cycle Protection)' '#SF009A_113' 'true' 'REQ:  SF009A_113' '' } %GIDa_90a6ce0b_65b8_4c4e_bf83_808cacb2e2cd"  TreatAsAtomicUnit=on
  CtrlTSelnEnabled : Subsystem  RequirementInfo="{'linktype_rmi_doors' '0000a52a (/E-STEER Core/SubSystem Specifications/Application Functions/SF009A Thermal Duty Cycle Protection)' '#SF009A_113' 'true' 'REQ:  SF009A_113' '' } %GIDa_5adee5c1_0f92_4e3b_a47a_20c823891ab9"  TreatAsAtomicUnit=on
  If1 : If  RequirementInfo="{'linktype_rmi_doors' '0000a52a (/E-STEER Core/SubSystem Specifications/Application Functions/SF009A Thermal Duty Cycle Protection)' '#SF009A_113' 'true' 'REQ:  SF009A_113' '' } %GIDa_0af20711_ed68_437a_866b_0dccaadd10e8"  IfExpression=u1
  Merge1 : Merge  RequirementInfo="{'linktype_rmi_doors' '0000a52a (/E-STEER Core/SubSystem Specifications/Application Functions/SF009A Thermal Duty Cycle Protection)' '#SF009A_113' 'true' 'REQ:  SF009A_113' '' } %GIDa_8e79fc40_c14e_47f4_a305_b8900f799e75"
  Mult12Temp : Outport
  wires:
  CtrlTSelnEnabled/1(Mult12) -> Merge1/1
  CtrlTSelnDisabled/1(Mult12) -> Merge1/2
  Merge1/1 -> Mult12Temp/1
  Calibration1/1 -> If1/1
  EcuTFild/1 -> CtrlTSelnEnabled/1(EcuTFild)
  MotFetT/1 -> CtrlTSelnDisabled/1(MotFetT)
  If1/1 -> CtrlTSelnEnabled/Action
  If1/2 -> CtrlTSelnDisabled/Action

== system SF009A_DutyCycThermProtn/DutyCycThermProtn/DutyCycThermProtnPer1/TemperatureSelection/Mult12T_DiagcStsLimdTPrfmncEnabled ==
  Action Port : ActionPort  ActionType=then
  Calibration : Constant  RequirementInfo="{'linktype_rmi_doors' '0000a52a (/E-STEER Core/SubSystem Specifications/Application Functions/SF009A Thermal Duty Cycle Protection)' '#SF009A_185' 'true' 'REQ:  SF009A_185' '' } %GIDa_7705fcc1_24c6_466a_9f03_d8760d1c7598"  Value=DutyCycThermProtnCtrlT
  CopyRight2 : Subsystem  Description=|  mask(Copyright Information){none=on}
      | Copyright info block.                                               
      |                                                                     
      | Place copyright information at the top of every subsystem in design.
      mask prompts: none "No parameters"
      mask help: Place copyright information at the top of every subsystem in design.
      mask Display:
      | NxtrConf = 'Nexteer Confidential';
      | 
      | sys = bdroot; %handle for the current model ("system")
      | first = get_param(sys,'Created');
      | first = first(end-3:end);  %year is last four digits
      | 
      | last = get_param(sys,'LastModifiedDate');
      | if isempty(last)
      |     last = datestr(now,'yyyy');
      | else
      |     last = last(end-3:end);
      | end
      | 
      | if strcmp(first,last)
      |     fprintf('%s -- Copyright %s Nexteer',NxtrConf,first)
      | else
      |     fprintf('%s -- %s%s- %s Nexteer',NxtrConf,char(169),first,last)
      | end
  Mult12Temp : Outport
  wires:
  Calibration/1 -> Mult12Temp/1
